simulink model "cla"  (R2015a)
settings: Solver=ode1  StartTime=0.0  StopTime=10.0  FixedStep=1  RelTol=1e-3
libraries: commutil2 x3
settings Model: Creator=Osmaz  LastModifiedBy=Osmaz

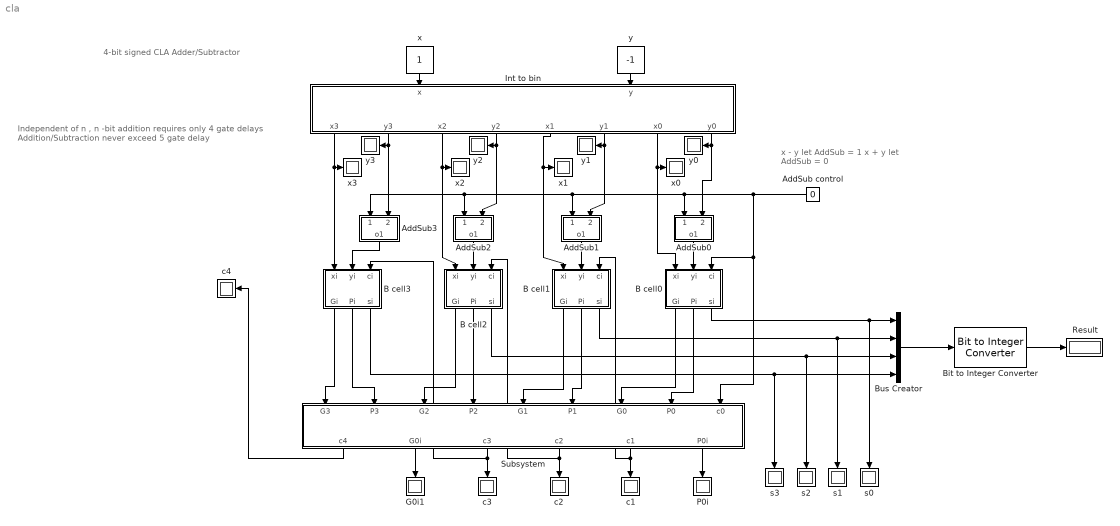
== system cla ==
  note: Independent of n ,
      | n -bit addition requires only 4 gate delays
      | Addition/Subtraction never exceed 5 gate delay
  note: 4-bit signed CLA Adder/Subtractor
  note: x - y let AddSub = 1
      | x + y let AddSub = 0
  AddSub control : Constant  Value=0  OutMin=0  OutMax=1  OutDataTypeStr=boolean
  AddSub0 : Subsystem
  AddSub1 : Subsystem
  AddSub2 : Subsystem
  AddSub3 : Subsystem
  B cell0 : Subsystem
  B cell1 : Subsystem
  B cell2 : Subsystem
  B cell3 : Subsystem
  Bit to Integer Converter : commutil2/Bit to Integer Converter  nbits=4  bitOrder=LSB first  signedOutputValues=Signed  outDtype=Inherit via internal rule  outDtypeSigned=Inherit via internal rule
  Bus Creator : BusCreator
  G0i1 : Display
  Int to bin : Subsystem
  P0i : Display
  Result : Display
  Subsystem : Subsystem
  c{1..4} (4 alike) : Display
  s{0..3} (4 alike) : Display
  x : Constant  OutMin=-8  OutMax=7  OutDataTypeStr=int8  SampleTime=1
  x{0..3} (4 alike) : Display
  y : Constant  Value=-1  OutMin=-8  OutMax=7  OutDataTypeStr=int8  SampleTime=1
  y{0..3} (4 alike) : Display
  wires:
  Int to bin/7(x0) -> x0/1, B cell0/1(xi)
  AddSub control/1 -> Subsystem/9(c0), B cell0/3(ci), AddSub0/1(1), AddSub1/1(1), AddSub3/1(1), AddSub2/1(1)
  Int to bin/5(x1) -> B cell1/1(xi), x1/1
  Int to bin/3(x2) -> B cell2/1(xi), x2/1
  Int to bin/1(x3) -> B cell3/1(xi), x3/1
  Bit to Integer Converter/1 -> Result/1
  Bus Creator/1 -> Bit to Integer Converter/1
  x/1 -> Int to bin/1(x)
  y/1 -> Int to bin/2(y)
  Int to bin/8(y0) -> AddSub0/2(2), y0/1
  Int to bin/6(y1) -> AddSub1/2(2), y1/1
  Int to bin/4(y2) -> y2/1, AddSub2/2(2)
  Int to bin/2(y3) -> AddSub3/2(2), y3/1
  AddSub1/1(o1) -> B cell1/2(yi)
  AddSub3/1(o1) -> B cell3/2(yi)
  B cell0/2(Pi) -> Subsystem/8(P0)
  B cell1/2(Pi) -> Subsystem/6(P1)
  B cell2/2(Pi) -> Subsystem/4(P2)
  B cell3/2(Pi) -> Subsystem/2(P3)
  B cell0/1(Gi) -> Subsystem/7(G0)
  B cell1/1(Gi) -> Subsystem/5(G1)
  B cell2/1(Gi) -> Subsystem/3(G2)
  B cell3/1(Gi) -> Subsystem/1(G3)
  Subsystem/5(c1) -> c1/1, B cell1/3(ci)
  Subsystem/4(c2) -> c2/1, B cell2/3(ci)
  Subsystem/1(c4) -> c4/1
  Subsystem/3(c3) -> B cell3/3(ci), c3/1
  B cell3/3(si) -> Bus Creator/4, s3/1
  B cell2/3(si) -> Bus Creator/3, s2/1
  B cell1/3(si) -> Bus Creator/2, s1/1
  B cell0/3(si) -> Bus Creator/1, s0/1
  AddSub0/1(o1) -> B cell0/2(yi)
  AddSub2/1(o1) -> B cell2/2(yi)
  Subsystem/6(P0i) -> P0i/1
  Subsystem/2(G0i) -> G0i1/1

== system cla/AddSub0 ==
  1 : Inport
  2 : Inport  Port=2
  Delay1 : Delay  DelayLength=1  InitialCondition=0  InputProcessing=Inherited
  XOR1 : Logic  Operator=XOR  IconShape=distinctive  AllPortsSameDT=off  OutDataTypeStr=boolean
  o1 : Outport
  wires:
  1/1 -> XOR1/2
  2/1 -> XOR1/1
  XOR1/1 -> Delay1/1
  Delay1/1 -> o1/1

== system cla/AddSub1 ==
  1 : Inport
  2 : Inport  Port=2
  Delay1 : Delay  DelayLength=1  InitialCondition=0  InputProcessing=Inherited
  XOR1 : Logic  Operator=XOR  IconShape=distinctive  AllPortsSameDT=off  OutDataTypeStr=boolean
  o1 : Outport
  wires:
  1/1 -> XOR1/2
  2/1 -> XOR1/1
  XOR1/1 -> Delay1/1
  Delay1/1 -> o1/1

== system cla/AddSub2 ==
  1 : Inport
  2 : Inport  Port=2
  Delay1 : Delay  DelayLength=1  InitialCondition=0  InputProcessing=Inherited
  XOR1 : Logic  Operator=XOR  IconShape=distinctive  AllPortsSameDT=off  OutDataTypeStr=boolean
  o1 : Outport
  wires:
  1/1 -> XOR1/2
  2/1 -> XOR1/1
  XOR1/1 -> Delay1/1
  Delay1/1 -> o1/1

== system cla/AddSub3 ==
  1 : Inport
  2 : Inport  Port=2
  Delay1 : Delay  DelayLength=1  InitialCondition=0  InputProcessing=Inherited
  XOR1 : Logic  Operator=XOR  IconShape=distinctive  AllPortsSameDT=off  OutDataTypeStr=boolean
  o1 : Outport
  wires:
  1/1 -> XOR1/2
  2/1 -> XOR1/1
  XOR1/1 -> Delay1/1
  Delay1/1 -> o1/1

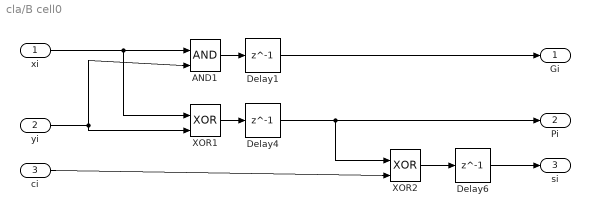
== system cla/B cell0 ==
  xi : Inport
  yi : Inport  Port=2
  ci : Inport  Port=3
  AND1 : Logic  IconShape=distinctive  AllPortsSameDT=off  OutDataTypeStr=boolean
  Delay1 : Delay  DelayLength=1  InitialCondition=0  InputProcessing=Inherited
  Delay4 : Delay  DelayLength=1  InitialCondition=0  InputProcessing=Inherited
  Delay6 : Delay  DelayLength=1  InitialCondition=0  InputProcessing=Inherited
  XOR1 : Logic  Operator=XOR  IconShape=distinctive  AllPortsSameDT=off  OutDataTypeStr=boolean
  XOR2 : Logic  Operator=XOR  IconShape=distinctive  AllPortsSameDT=off  OutDataTypeStr=boolean
  Gi : Outport
  Pi : Outport  Port=2
  si : Outport  Port=3
  wires:
  AND1/1 -> Delay1/1
  yi/1 -> AND1/2, XOR1/2
  xi/1 -> AND1/1, XOR1/1
  ci/1 -> XOR2/2
  Delay1/1 -> Gi/1
  Delay6/1 -> si/1
  XOR1/1 -> Delay4/1
  Delay4/1 -> Pi/1, XOR2/1
  XOR2/1 -> Delay6/1

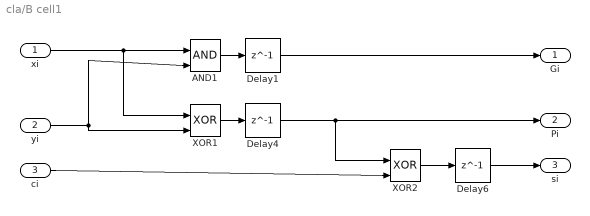
== system cla/B cell1 ==
  xi : Inport
  yi : Inport  Port=2
  ci : Inport  Port=3
  AND1 : Logic  IconShape=distinctive  AllPortsSameDT=off  OutDataTypeStr=boolean
  Delay1 : Delay  DelayLength=1  InitialCondition=0  InputProcessing=Inherited
  Delay4 : Delay  DelayLength=1  InitialCondition=0  InputProcessing=Inherited
  Delay6 : Delay  DelayLength=1  InitialCondition=0  InputProcessing=Inherited
  XOR1 : Logic  Operator=XOR  IconShape=distinctive  AllPortsSameDT=off  OutDataTypeStr=boolean
  XOR2 : Logic  Operator=XOR  IconShape=distinctive  AllPortsSameDT=off  OutDataTypeStr=boolean
  Gi : Outport
  Pi : Outport  Port=2
  si : Outport  Port=3
  wires:
  AND1/1 -> Delay1/1
  yi/1 -> AND1/2, XOR1/2
  xi/1 -> AND1/1, XOR1/1
  ci/1 -> XOR2/2
  Delay1/1 -> Gi/1
  Delay6/1 -> si/1
  XOR1/1 -> Delay4/1
  Delay4/1 -> Pi/1, XOR2/1
  XOR2/1 -> Delay6/1

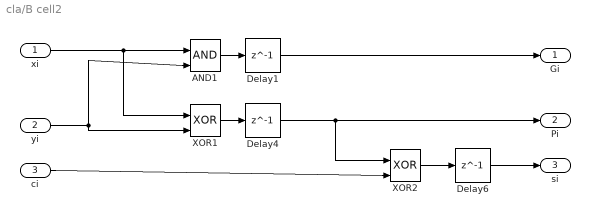
== system cla/B cell2 ==
  xi : Inport
  yi : Inport  Port=2
  ci : Inport  Port=3
  AND1 : Logic  IconShape=distinctive  AllPortsSameDT=off  OutDataTypeStr=boolean
  Delay1 : Delay  DelayLength=1  InitialCondition=0  InputProcessing=Inherited
  Delay4 : Delay  DelayLength=1  InitialCondition=0  InputProcessing=Inherited
  Delay6 : Delay  DelayLength=1  InitialCondition=0  InputProcessing=Inherited
  XOR1 : Logic  Operator=XOR  IconShape=distinctive  AllPortsSameDT=off  OutDataTypeStr=boolean
  XOR2 : Logic  Operator=XOR  IconShape=distinctive  AllPortsSameDT=off  OutDataTypeStr=boolean
  Gi : Outport
  Pi : Outport  Port=2
  si : Outport  Port=3
  wires:
  AND1/1 -> Delay1/1
  yi/1 -> AND1/2, XOR1/2
  xi/1 -> AND1/1, XOR1/1
  ci/1 -> XOR2/2
  Delay1/1 -> Gi/1
  Delay6/1 -> si/1
  XOR1/1 -> Delay4/1
  Delay4/1 -> Pi/1, XOR2/1
  XOR2/1 -> Delay6/1

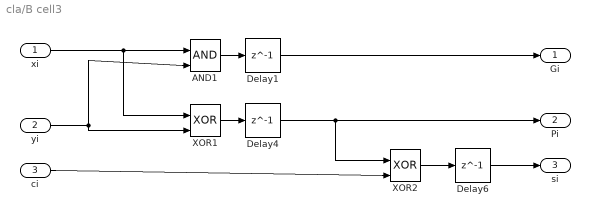
== system cla/B cell3 ==
  xi : Inport
  yi : Inport  Port=2
  ci : Inport  Port=3
  AND1 : Logic  IconShape=distinctive  AllPortsSameDT=off  OutDataTypeStr=boolean
  Delay1 : Delay  DelayLength=1  InitialCondition=0  InputProcessing=Inherited
  Delay4 : Delay  DelayLength=1  InitialCondition=0  InputProcessing=Inherited
  Delay6 : Delay  DelayLength=1  InitialCondition=0  InputProcessing=Inherited
  XOR1 : Logic  Operator=XOR  IconShape=distinctive  AllPortsSameDT=off  OutDataTypeStr=boolean
  XOR2 : Logic  Operator=XOR  IconShape=distinctive  AllPortsSameDT=off  OutDataTypeStr=boolean
  Gi : Outport
  Pi : Outport  Port=2
  si : Outport  Port=3
  wires:
  AND1/1 -> Delay1/1
  yi/1 -> AND1/2, XOR1/2
  xi/1 -> AND1/1, XOR1/1
  ci/1 -> XOR2/2
  Delay1/1 -> Gi/1
  Delay6/1 -> si/1
  XOR1/1 -> Delay4/1
  Delay4/1 -> Pi/1, XOR2/1
  XOR2/1 -> Delay6/1

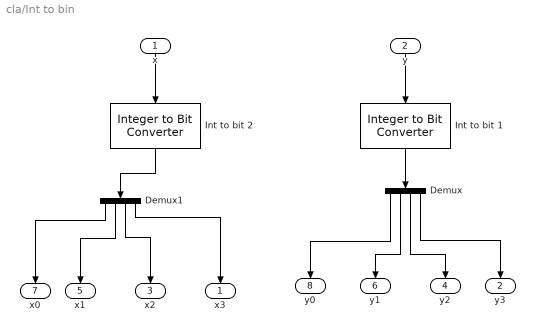
== system cla/Int to bin ==
  x : Inport
  y : Inport  Port=2
  Demux : Demux
  Demux1 : Demux
  Int to bit 1 : commutil2/Integer to Bit Converter  nbits=4  signedInputValues=Signed  bitOrder=LSB first  outDtype=Inherit via internal rule
  Int to bit 2 : commutil2/Integer to Bit Converter  nbits=4  signedInputValues=Signed  bitOrder=LSB first  outDtype=Inherit via internal rule
  x3 : Outport
  y3 : Outport  Port=2
  x2 : Outport  Port=3
  y2 : Outport  Port=4
  x1 : Outport  Port=5
  y1 : Outport  Port=6
  x0 : Outport  Port=7
  y0 : Outport  Port=8
  wires:
  Demux1/1 -> x0/1
  Demux/2 -> y1/1
  Demux1/2 -> x1/1
  Demux/1 -> y0/1
  y/1 -> Int to bit 1/1
  Int to bit 1/1 -> Demux/1
  x/1 -> Int to bit 2/1
  Demux1/3 -> x2/1
  Demux1/4 -> x3/1
  Demux/3 -> y2/1
  Int to bit 2/1 -> Demux1/1
  Demux/4 -> y3/1

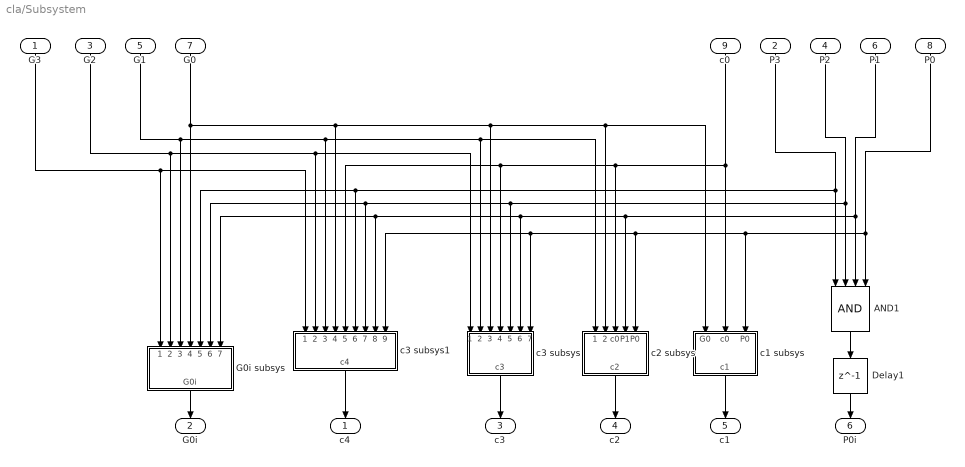
== system cla/Subsystem ==
  G3 : Inport
  P3 : Inport  Port=2
  G2 : Inport  Port=3
  P2 : Inport  Port=4
  G1 : Inport  Port=5
  P1 : Inport  Port=6
  G0 : Inport  Port=7
  P0 : Inport  Port=8
  c0 : Inport  Port=9
  AND1 : Logic  Inputs=4  IconShape=distinctive  AllPortsSameDT=off  OutDataTypeStr=boolean
  Delay1 : Delay  DelayLength=1  InitialCondition=0  InputProcessing=Inherited
  G0i subsys : Subsystem
  c1 subsys : Subsystem
  c2 subsys : Subsystem
  c3 subsys : Subsystem
  c3 subsys1 : Subsystem
  c4 : Outport
  G0i : Outport  Port=2
  c3 : Outport  Port=3
  c2 : Outport  Port=4
  c1 : Outport  Port=5
  P0i : Outport  Port=6
  wires:
  G0i subsys/1(G0i) -> G0i/1
  P2/1 -> G0i subsys/6(P2), c3 subsys1/7(P2), c3 subsys/5(P2), AND1/2
  P3/1 -> G0i subsys/5(P3), c3 subsys1/6(P3), AND1/1
  G3/1 -> c3 subsys1/1(G3), G0i subsys/1(G3)
  AND1/1 -> Delay1/1
  Delay1/1 -> P0i/1
  c0/1 -> c2 subsys/3(c0), c3 subsys1/5(c0), c3 subsys/4(c0), c1 subsys/2(c0)
  P0/1 -> AND1/4, c3 subsys1/9(P0), c3 subsys/7(P0), c2 subsys/5(P0), c1 subsys/3(P0)
  c1 subsys/1(c1) -> c1/1
  G0/1 -> c3 subsys1/4(G0), c3 subsys/3(G0), c2 subsys/2(G0), c1 subsys/1(G0), G0i subsys/4(G0)
  G1/1 -> c3 subsys1/3(G1), c3 subsys/2(G1), c2 subsys/1(G1), G0i subsys/3(G1)
  c2 subsys/1(c2) -> c2/1
  P1/1 -> G0i subsys/7(P1), c3 subsys1/8(P1), c3 subsys/6(P1), c2 subsys/4(P1), AND1/3
  c3 subsys/1(c3) -> c3/1
  G2/1 -> c3 subsys1/2(G2), c3 subsys/1(G2), G0i subsys/2(G2)
  c3 subsys1/1(c4) -> c4/1

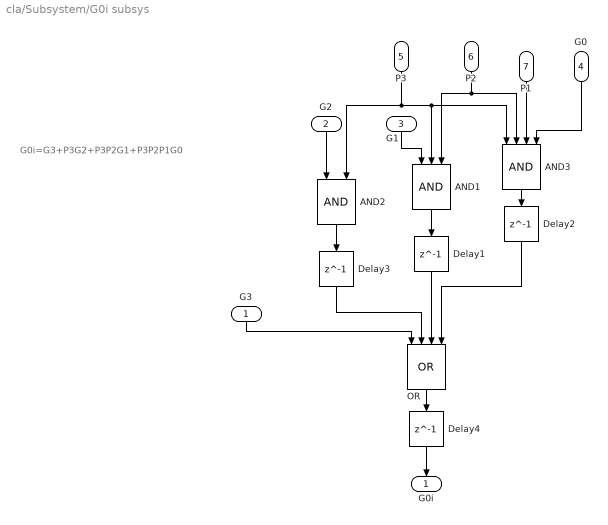
== system cla/Subsystem/G0i subsys ==
  note: G0i=G3+P3G2+P3P2G1+P3P2P1G0
  G3 : Inport
  G2 : Inport  Port=2
  G1 : Inport  Port=3
  G0 : Inport  Port=4
  P3 : Inport  Port=5
  P2 : Inport  Port=6
  P1 : Inport  Port=7
  AND1 : Logic  Inputs=3  IconShape=distinctive  AllPortsSameDT=off  OutDataTypeStr=boolean
  AND2 : Logic  IconShape=distinctive  AllPortsSameDT=off  OutDataTypeStr=boolean
  AND3 : Logic  Inputs=4  IconShape=distinctive  AllPortsSameDT=off  OutDataTypeStr=boolean
  Delay{1..4} (4 alike) : Delay  DelayLength=1  InitialCondition=0  InputProcessing=Inherited
  OR : Logic  Operator=OR  Inputs=4  IconShape=distinctive  AllPortsSameDT=off  OutDataTypeStr=boolean
  G0i : Outport
  wires:
  OR/1 -> Delay4/1
  Delay4/1 -> G0i/1
  AND3/1 -> Delay2/1
  Delay2/1 -> OR/4
  P2/1 -> AND3/2, AND1/3
  Delay1/1 -> OR/3
  AND1/1 -> Delay1/1
  G1/1 -> AND1/1
  G0/1 -> AND3/4
  P1/1 -> AND3/3
  P3/1 -> AND1/2, AND3/1, AND2/2
  G2/1 -> AND2/1
  AND2/1 -> Delay3/1
  Delay3/1 -> OR/2
  G3/1 -> OR/1

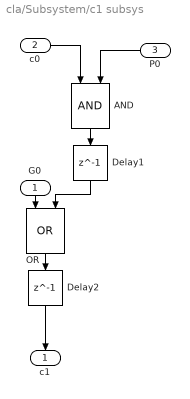
== system cla/Subsystem/c1 subsys ==
  G0 : Inport
  c0 : Inport  Port=2
  P0 : Inport  Port=3
  AND : Logic  IconShape=distinctive  AllPortsSameDT=off  OutDataTypeStr=boolean
  Delay1 : Delay  DelayLength=1  InitialCondition=0  InputProcessing=Inherited
  Delay2 : Delay  DelayLength=1  InitialCondition=0  InputProcessing=Inherited
  OR : Logic  Operator=OR  IconShape=distinctive  AllPortsSameDT=off  OutDataTypeStr=boolean
  c1 : Outport
  wires:
  OR/1 -> Delay2/1
  Delay2/1 -> c1/1
  AND/1 -> Delay1/1
  Delay1/1 -> OR/2
  c0/1 -> AND/1
  G0/1 -> OR/1
  P0/1 -> AND/2

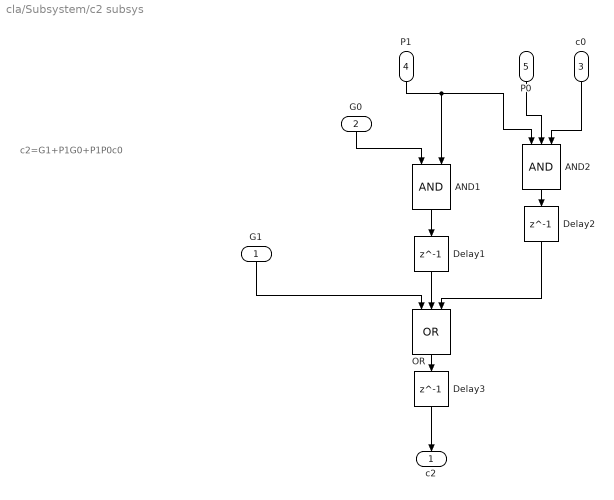
== system cla/Subsystem/c2 subsys ==
  note: c2=G1+P1G0+P1P0c0
  G1 : Inport
  G0 : Inport  Port=2
  c0 : Inport  Port=3
  P1 : Inport  Port=4
  P0 : Inport  Port=5
  AND1 : Logic  IconShape=distinctive  AllPortsSameDT=off  OutDataTypeStr=boolean
  AND2 : Logic  Inputs=3  IconShape=distinctive  AllPortsSameDT=off  OutDataTypeStr=boolean
  Delay1 : Delay  DelayLength=1  InitialCondition=0  InputProcessing=Inherited
  Delay2 : Delay  DelayLength=1  InitialCondition=0  InputProcessing=Inherited
  Delay3 : Delay  DelayLength=1  InitialCondition=0  InputProcessing=Inherited
  OR : Logic  Operator=OR  Inputs=3  IconShape=distinctive  AllPortsSameDT=off  OutDataTypeStr=boolean
  c2 : Outport
  wires:
  OR/1 -> Delay3/1
  Delay3/1 -> c2/1
  AND2/1 -> Delay2/1
  G1/1 -> OR/1
  Delay2/1 -> OR/3
  c0/1 -> AND2/3
  P0/1 -> AND2/2
  P1/1 -> AND1/2, AND2/1
  Delay1/1 -> OR/2
  AND1/1 -> Delay1/1
  G0/1 -> AND1/1

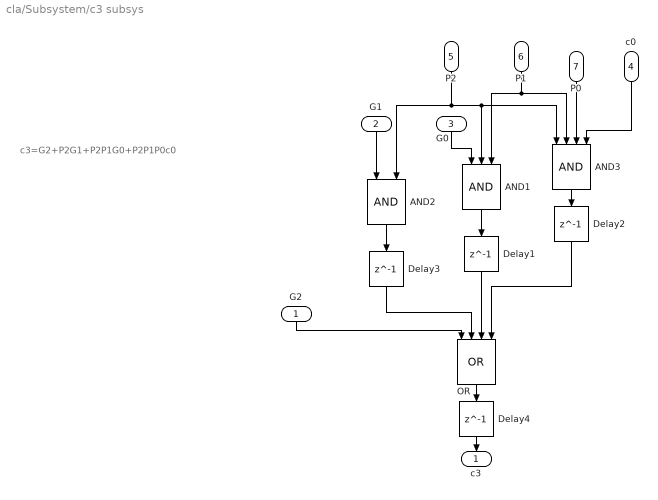
== system cla/Subsystem/c3 subsys ==
  note: c3=G2+P2G1+P2P1G0+P2P1P0c0
  G2 : Inport
  G1 : Inport  Port=2
  G0 : Inport  Port=3
  c0 : Inport  Port=4
  P2 : Inport  Port=5
  P1 : Inport  Port=6
  P0 : Inport  Port=7
  AND1 : Logic  Inputs=3  IconShape=distinctive  AllPortsSameDT=off  OutDataTypeStr=boolean
  AND2 : Logic  IconShape=distinctive  AllPortsSameDT=off  OutDataTypeStr=boolean
  AND3 : Logic  Inputs=4  IconShape=distinctive  AllPortsSameDT=off  OutDataTypeStr=boolean
  Delay{1..4} (4 alike) : Delay  DelayLength=1  InitialCondition=0  InputProcessing=Inherited
  OR : Logic  Operator=OR  Inputs=4  IconShape=distinctive  AllPortsSameDT=off  OutDataTypeStr=boolean
  c3 : Outport
  wires:
  OR/1 -> Delay4/1
  Delay4/1 -> c3/1
  AND3/1 -> Delay2/1
  Delay2/1 -> OR/4
  P1/1 -> AND3/2, AND1/3
  Delay1/1 -> OR/3
  AND1/1 -> Delay1/1
  G0/1 -> AND1/1
  c0/1 -> AND3/4
  P0/1 -> AND3/3
  P2/1 -> AND1/2, AND3/1, AND2/2
  G1/1 -> AND2/1
  AND2/1 -> Delay3/1
  Delay3/1 -> OR/2
  G2/1 -> OR/1

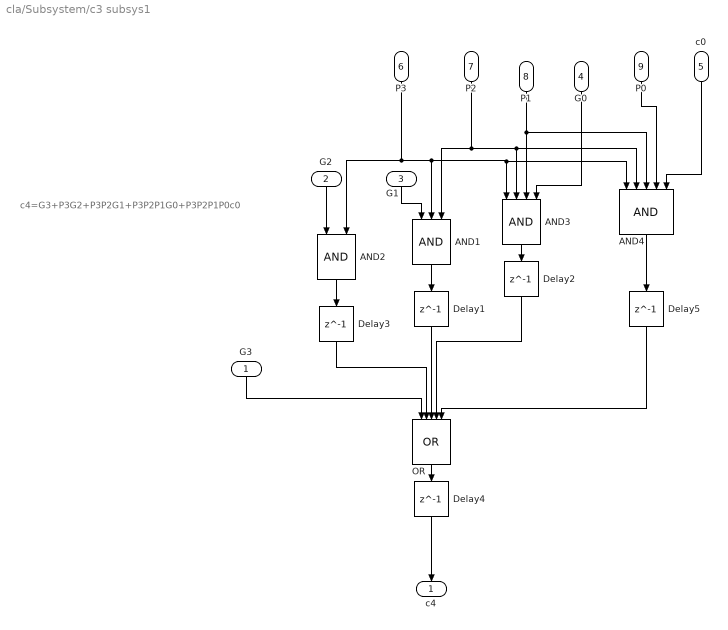
== system cla/Subsystem/c3 subsys1 ==
  note: c4=G3+P3G2+P3P2G1+P3P2P1G0+P3P2P1P0c0
  G3 : Inport
  G2 : Inport  Port=2
  G1 : Inport  Port=3
  G0 : Inport  Port=4
  c0 : Inport  Port=5
  P3 : Inport  Port=6
  P2 : Inport  Port=7
  P1 : Inport  Port=8
  P0 : Inport  Port=9
  AND1 : Logic  Inputs=3  IconShape=distinctive  AllPortsSameDT=off  OutDataTypeStr=boolean
  AND2 : Logic  IconShape=distinctive  AllPortsSameDT=off  OutDataTypeStr=boolean
  AND3 : Logic  Inputs=4  IconShape=distinctive  AllPortsSameDT=off  OutDataTypeStr=boolean
  AND4 : Logic  Inputs=5  IconShape=distinctive  AllPortsSameDT=off  OutDataTypeStr=boolean
  Delay{1..5} (5 alike) : Delay  DelayLength=1  InitialCondition=0  InputProcessing=Inherited
  OR : Logic  Operator=OR  Inputs=5  IconShape=distinctive  AllPortsSameDT=off  OutDataTypeStr=boolean
  c4 : Outport
  wires:
  OR/1 -> Delay4/1
  Delay4/1 -> c4/1
  AND3/1 -> Delay2/1
  Delay2/1 -> OR/4
  P2/1 -> AND4/2, AND3/2, AND1/3
  Delay1/1 -> OR/3
  AND1/1 -> Delay1/1
  G1/1 -> AND1/1
  G0/1 -> AND3/4
  P1/1 -> AND4/3, AND3/3
  P3/1 -> AND1/2, AND4/1, AND3/1, AND2/2
  G2/1 -> AND2/1
  AND2/1 -> Delay3/1
  Delay3/1 -> OR/2
  G3/1 -> OR/1
  P0/1 -> AND4/4
  c0/1 -> AND4/5
  Delay5/1 -> OR/5
  AND4/1 -> Delay5/1
